simulink model "OMAP"  (R2018b)
settings: Solver=FixedStepDiscrete  StartTime=0.0  StopTime=10.0  FixedStep=0.01  RelTol=1e-3
values from neighbouring files (symbols this model uses):
  Clb_ICADirect_LaneDisp_StateFive = Simulink.Parameter    [omap_ver_442.m]
  Clb_ICADirect_LaneDisp_StateFour = Simulink.Parameter    [omap_ver_442.m]
  Clb_ICADirect_LaneDisp_StateOne = Simulink.Parameter    [omap_ver_442.m]
  Clb_ICADirect_LaneDisp_StateThree = Simulink.Parameter    [omap_ver_442.m]
  Clb_ICADirect_LaneDisp_StateTwo = Simulink.Parameter    [omap_ver_442.m]
  Clb_ICADirect_LaneDisp_StateZero = Simulink.Parameter    [omap_ver_442.m]
  Clb_ICADirect_LaneDispSW = Simulink.Parameter    [omap_ver_442.m]
  Clb_ICADirect_TrnLghtsCom_Switch = Simulink.Parameter    [omap_ver_442.m]
  Clb_ICADirect_TrnLghtsCom_Value = Simulink.Parameter    [omap_ver_442.m]
  Clb_ICADirect_TrnLghtsCrtl_Inhb = Simulink.Parameter    [omap_ver_442.m]
  OMAP_ACCAEB_EMSESC_Decel = Simulink.Parameter    [omap_ver_442.m]
  OMAP_ACCFCW_IC_Decel = Simulink.Parameter    [omap_ver_442.m]
  OMAP_clb_ACC_RVVReqType = Simulink.Parameter    [omap_ver_442.m]
  OMAP_clb_ACC_RVVReqType_Switch = Simulink.Parameter    [omap_ver_442.m]
  OMAP_clb_ACCHeadwayDisplay = Simulink.Parameter    [omap_ver_442.m]
  OMAP_clb_ACCHeadwayDisplay_Switch = Simulink.Parameter    [omap_ver_442.m]
  OMAP_clb_ACCHeadwayIcon = Simulink.Parameter    [omap_ver_442.m]
  OMAP_clb_ACCHeadwayIcon_Switch = Simulink.Parameter    [omap_ver_442.m]
  OMAP_clb_ACCMessagePrompt = Simulink.Parameter    [omap_ver_442.m]
  OMAP_clb_ACCMessagePrompt_Switch = Simulink.Parameter    [omap_ver_442.m]
  OMAP_clb_ACCRequestEPB = Simulink.Parameter    [omap_ver_442.m]
  OMAP_clb_ACCRequestEPB_Switch = Simulink.Parameter    [omap_ver_442.m]
  OMAP_clb_ACCSetSpeed = Simulink.Parameter    [omap_ver_442.m]
  OMAP_clb_ACCSetSpeed_Switch = Simulink.Parameter    [omap_ver_442.m]
  OMAP_clb_ACCSetSpeedDis = Simulink.Parameter    [omap_ver_442.m]
  OMAP_clb_ACCSetSpeedDis_Switch = Simulink.Parameter    [omap_ver_442.m]
  OMAP_clb_ACCState = Simulink.Parameter    [omap_ver_442.m]
  OMAP_clb_ACCState_Switch = Simulink.Parameter    [omap_ver_442.m]
  OMAP_clb_ACCStatusIconDis = Simulink.Parameter    [omap_ver_442.m]
  OMAP_clb_ACCStatusIconDis_Switch = Simulink.Parameter    [omap_ver_442.m]
  OMAP_clb_ACCTorqueReq = Simulink.Parameter    [omap_ver_442.m]
  OMAP_clb_ACCTorqueReq_Switch = Simulink.Parameter    [omap_ver_442.m]
  OMAP_clb_ADAS_State = Simulink.Parameter    [omap_ver_442.m]
  OMAP_clb_ADAS_State_Switch = Simulink.Parameter    [omap_ver_442.m]
  OMAP_clb_AEBAlertReq = Simulink.Parameter    [omap_ver_442.m]
  OMAP_clb_AEBAlertReq_Switch = Simulink.Parameter    [omap_ver_442.m]
  OMAP_clb_AEBBrakingProg = Simulink.Parameter    [omap_ver_442.m]
  OMAP_clb_AEBBrakingProg_Switch = Simulink.Parameter    [omap_ver_442.m]
  OMAP_clb_AEBFaultStatus = Simulink.Parameter    [omap_ver_442.m]
  OMAP_clb_AEBFaultStatus_Switch = Simulink.Parameter    [omap_ver_442.m]
  OMAP_clb_AEBMassageDisp = Simulink.Parameter    [omap_ver_442.m]
  OMAP_clb_AEBMassageDisp_Switch = Simulink.Parameter    [omap_ver_442.m]
  OMAP_clb_AEBState = Simulink.Parameter    [omap_ver_442.m]
  OMAP_clb_AEBState_Switch = Simulink.Parameter    [omap_ver_442.m]
  OMAP_clb_AEBSwitchStatus = Simulink.Parameter    [omap_ver_442.m]
  OMAP_clb_AEBSwitchStatus_Switch = Simulink.Parameter    [omap_ver_442.m]
  OMAP_clb_BrakeRequest = Simulink.Parameter    [omap_ver_442.m]
  OMAP_clb_BrakeRequest_Switch = Simulink.Parameter    [omap_ver_442.m]
  OMAP_clb_DecelerationSet = Simulink.Parameter    [omap_ver_442.m]
  OMAP_clb_DecelerationSet_Switch = Simulink.Parameter    [omap_ver_442.m]
  OMAP_clb_DecelerationType = Simulink.Parameter    [omap_ver_442.m]
  OMAP_clb_DecelerationType_Switch = Simulink.Parameter    [omap_ver_442.m]
  OMAP_clb_DeclControlReq = Simulink.Parameter    [omap_ver_442.m]
  OMAP_clb_DeclControlReq_Switch = Simulink.Parameter    [omap_ver_442.m]
  OMAP_clb_DownorUpGearMinTime = Simulink.Parameter    [omap_ver_442.m]
  OMAP_clb_DownorUpGearMinTime_Switch = Simulink.Parameter    [omap_ver_442.m]
  OMAP_clb_ELKPopupMessage = Simulink.Parameter    [omap_ver_442.m]
  OMAP_clb_ELKPopupMessage_Switch = Simulink.Parameter    [omap_ver_442.m]
  OMAP_clb_ELKSts = Simulink.Parameter    [omap_ver_442.m]
  OMAP_clb_ELKSts_Switch = Simulink.Parameter    [omap_ver_442.m]
  OMAP_clb_ESAFaultSt = Simulink.Parameter    [omap_ver_442.m]
  OMAP_clb_ESAFaultSt_Switch = Simulink.Parameter    [omap_ver_442.m]
  OMAP_clb_ESARequest = Simulink.Parameter    [omap_ver_442.m]
  OMAP_clb_ESARequest_Switch = Simulink.Parameter    [omap_ver_442.m]
  OMAP_clb_ESAState = Simulink.Parameter    [omap_ver_442.m]
  OMAP_clb_ESAState_Switch = Simulink.Parameter    [omap_ver_442.m]
  OMAP_clb_ESATorqueReq = Simulink.Parameter    [omap_ver_442.m]
  OMAP_clb_ESATorqueReq_Switch = Simulink.Parameter    [omap_ver_442.m]
  OMAP_clb_ESCDriveOff = Simulink.Parameter    [omap_ver_442.m]
  OMAP_clb_ESCDriveOff_Switch = Simulink.Parameter    [omap_ver_442.m]
  OMAP_clb_ESCHoldReq = Simulink.Parameter    [omap_ver_442.m]
  OMAP_clb_ESCHoldReq_Switch = Simulink.Parameter    [omap_ver_442.m]
  OMAP_clb_Handsoffwarning = Simulink.Parameter    [omap_ver_442.m]
  OMAP_clb_Handsoffwarning_Switch = Simulink.Parameter    [omap_ver_442.m]
  OMAP_clb_HapticAlarmReq = Simulink.Parameter    [omap_ver_442.m]
  OMAP_clb_HapticAlarmReq_Switch = Simulink.Parameter    [omap_ver_442.m]
  OMAP_clb_HMIPopupMassage = Simulink.Parameter    [omap_ver_442.m]
  OMAP_clb_HMIPopupMassage_Switch = Simulink.Parameter    [omap_ver_442.m]
  OMAP_clb_HWAActionSts = Simulink.Parameter    [omap_ver_442.m]
  OMAP_clb_HWAActionSts_Switch = Simulink.Parameter    [omap_ver_442.m]
  OMAP_clb_HWAMode = Simulink.Parameter    [omap_ver_442.m]
  OMAP_clb_HWAMode_Switch = Simulink.Parameter    [omap_ver_442.m]
  OMAP_clb_HWATurnOnIdctr = Simulink.Parameter    [omap_ver_442.m]
  OMAP_clb_HWATurnOnIdctr_Switch = Simulink.Parameter    [omap_ver_442.m]
  OMAP_clb_ICAMassageDisp = Simulink.Parameter    [omap_ver_442.m]
  OMAP_clb_ICAMassageDisp_Switch = Simulink.Parameter    [omap_ver_442.m]
  OMAP_clb_ICAStatusIcon = Simulink.Parameter    [omap_ver_442.m]
  OMAP_clb_ICAStatusIcon_Switch = Simulink.Parameter    [omap_ver_442.m]
  OMAP_clb_ISLCDriverRemind = Simulink.Parameter    [omap_ver_442.m]
  OMAP_clb_ISLCDriverRemind_Switch = Simulink.Parameter    [omap_ver_442.m]
  OMAP_clb_ISLCState = Simulink.Parameter    [omap_ver_442.m]
  OMAP_clb_ISLCState_Switch = Simulink.Parameter    [omap_ver_442.m]
  OMAP_clb_JAFaultSt = Simulink.Parameter    [omap_ver_442.m]
  OMAP_clb_JAFaultSt_Switch = Simulink.Parameter    [omap_ver_442.m]
  OMAP_clb_LCAPopupMessage = Simulink.Parameter    [omap_ver_442.m]
  OMAP_clb_LCAPopupMessage_Switch = Simulink.Parameter    [omap_ver_442.m]
  OMAP_clb_LCAStatusDisplay = Simulink.Parameter    [omap_ver_442.m]
  OMAP_clb_LCAStatusDisplay_Switch = Simulink.Parameter    [omap_ver_442.m]
  OMAP_clb_LDWStatusDisplay = Simulink.Parameter    [omap_ver_442.m]
  OMAP_clb_LDWStatusDisplay_Switch = Simulink.Parameter    [omap_ver_442.m]
  OMAP_clb_LDWWarningSt = Simulink.Parameter    [omap_ver_442.m]
  OMAP_clb_LDWWarningSt_Switch = Simulink.Parameter    [omap_ver_442.m]
  OMAP_clb_LightControlValid = Simulink.Parameter    [omap_ver_442.m]
  OMAP_clb_LightControlValid_Switch = Simulink.Parameter    [omap_ver_442.m]
  OMAP_clb_LKAActivation = Simulink.Parameter    [omap_ver_442.m]
  OMAP_clb_LKAActivation_Switch = Simulink.Parameter    [omap_ver_442.m]
  OMAP_clb_LKAAngleReq = Simulink.Parameter    [omap_ver_442.m]
  OMAP_clb_LKAAngleReq_Switch = Simulink.Parameter    [omap_ver_442.m]
  OMAP_clb_LKAMode = Simulink.Parameter    [omap_ver_442.m]
  OMAP_clb_LKAMode_Switch = Simulink.Parameter    [omap_ver_442.m]
  OMAP_clb_LKAorELK_CoolTime = Simulink.Parameter    [omap_ver_442.m]
  OMAP_clb_LKAState = Simulink.Parameter    [omap_ver_442.m]
  OMAP_clb_LKAState_Switch = Simulink.Parameter    [omap_ver_442.m]
  OMAP_clb_LKAStatusDisplay = Simulink.Parameter    [omap_ver_442.m]
  OMAP_clb_LKAStatusDisplay_Switch = Simulink.Parameter    [omap_ver_442.m]
  OMAP_clb_LKASwitchState = Simulink.Parameter    [omap_ver_442.m]
  OMAP_clb_LKASwitchState_Switch = Simulink.Parameter    [omap_ver_442.m]
  OMAP_clb_LKATorqFactReq = Simulink.Parameter    [omap_ver_442.m]
  OMAP_clb_LKATorqFactReq_Switch = Simulink.Parameter    [omap_ver_442.m]
  OMAP_clb_PrefillRequest = Simulink.Parameter    [omap_ver_442.m]
  ... (+36 more)
libraries: simulink x184, canmsglib x2
(part 2 of 14)

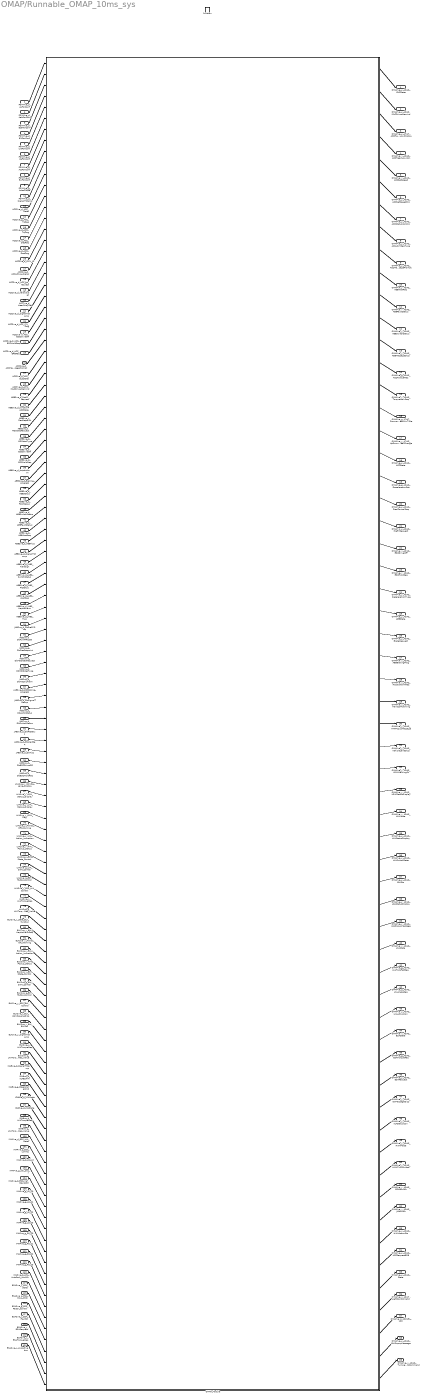
== system OMAP/Runnable_OMAP_10ms_sys ==
  FDMMve_d_JaFcnConf : Inport  OutDataTypeStr=uint16  PortDimensions=1
  FDMMve_d_AebFcnConf : Inport  Port=2  OutDataTypeStr=uint16  PortDimensions=1
  FDMMve_d_EsaFcnConf : Inport  Port=3  OutDataTypeStr=uint16  PortDimensions=1
  FDMMve_d_ElkFcnConf : Inport  Port=4  OutDataTypeStr=uint16  PortDimensions=1
  FDMMve_d_LkaFcnConf : Inport  Port=5  OutDataTypeStr=uint16  PortDimensions=1
  FDMMve_d_IcaFcnConf : Inport  Port=6  OutDataTypeStr=uint16  PortDimensions=1
  FDMMve_d_AccFcnConf : Inport  Port=7  OutDataTypeStr=uint16  PortDimensions=1
  FDMMve_d_EwFcnConf : Inport  Port=8  OutDataTypeStr=uint16  PortDimensions=1
  FDMMve_g_Adas2Fapa : Inport  Port=9  OutDataTypeStr=uint32  PortDimensions=1
  FDMMve_d_SignalTStamp : Inport  Port=10  OutDataTypeStr=uint16  PortDimensions=1
  ACCSve_d_ACC_State : Inport  Port=11  OutDataTypeStr=uint16  PortDimensions=1
  ACCSve_g_ACC_TqReq : Inport  Port=12  OutDataTypeStr=single  PortDimensions=1
  ACCSve_d_ACC_TqFlag : Inport  Port=13  OutDataTypeStr=uint16  PortDimensions=1
  ACCSve_g_ACC_DecReq : Inport  Port=14  OutDataTypeStr=single  PortDimensions=1
  ACCSve_d_ACC_DecFlag : Inport  Port=15  OutDataTypeStr=uint16  PortDimensions=1
  ACCSve_d_CIPV_ID : Inport  Port=16  OutDataTypeStr=uint16  PortDimensions=1
  ACCSve_d_ACCActive_Signal : Inport  Port=17  OutDataTypeStr=uint16  PortDimensions=1
  ACCSve_d_ACC_go_request : Inport  Port=18  OutDataTypeStr=uint16  PortDimensions=1
  ACCSve_d_VelocitySet : Inport  Port=19  OutDataTypeStr=uint16  PortDimensions=1
  ACCSve_d_HeadWaySet : Inport  Port=20  OutDataTypeStr=uint16  PortDimensions=1
  ACCSve_d_SignalTStamp : Inport  Port=21  OutDataTypeStr=uint16  PortDimensions=1
  ACCSve_d_ACC_ICA_Flag : Inport  Port=22  OutDataTypeStr=uint16  PortDimensions=1
  ACCSve_d_ACC_ESCDriveOff : Inport  Port=23  OutDataTypeStr=uint16  PortDimensions=1
  ACCSve_d_ACC_ESCHoldReq : Inport  Port=24  OutDataTypeStr=uint16  PortDimensions=1
  ACCSve_d_ACC_EPBReq : Inport  Port=25  OutDataTypeStr=uint16  PortDimensions=1
  ACCSve_d_ACCMessagePrompt : Inport  Port=26  OutDataTypeStr=uint16
  ACCSve_d_ACC_ISLCState : Inport  Port=27  OutDataTypeStr=uint16  PortDimensions=1
  ACCSve_d_ACC_ISLCDriverRemind : Inport  Port=28  OutDataTypeStr=uint16  PortDimensions=1
  AEBSve_d_Prefill_request : Inport  Port=29  OutDataTypeStr=uint16  PortDimensions=1
  AEBSve_d_functionFARCState : Inport  Port=30  OutDataTypeStr=uint16  PortDimensions=1
  AEBSve_g_DecSetpoint : Inport  Port=31  OutDataTypeStr=single  PortDimensions=1
  AEBSve_d_MDDdecRequest : Inport  Port=32  OutDataTypeStr=uint16  PortDimensions=1
  AEBSve_d_MDDdecType : Inport  Port=33  OutDataTypeStr=uint16  PortDimensions=1
  AEBSve_d_ESCDriveOff : Inport  Port=34  OutDataTypeStr=uint16  PortDimensions=1
  AEBSve_d_ESCHoldReq : Inport  Port=35  OutDataTypeStr=uint16  PortDimensions=1
  AEBSve_d_HapticAlarm : Inport  Port=36  OutDataTypeStr=uint16  PortDimensions=1
  AEBSve_d_Braking_progress : Inport  Port=37  OutDataTypeStr=uint16  PortDimensions=1
  AEBSve_d_AEBStatus : Inport  Port=38  OutDataTypeStr=uint16  PortDimensions=1
  AEBSve_d_FCWStatus : Inport  Port=39  OutDataTypeStr=uint16  PortDimensions=1
  AEBSve_d_AEBSwitchStatus : Inport  Port=40  OutDataTypeStr=uint16  PortDimensions=1
  AEBSve_d_AEBFaultStatus : Inport  Port=41  OutDataTypeStr=uint16  PortDimensions=1
  AEBSve_d_AEBAlertReq : Inport  Port=42  OutDataTypeStr=uint16  PortDimensions=1
  AEBSve_d_AEBTips : Inport  Port=43  OutDataTypeStr=uint16  PortDimensions=1
  AEBSve_d_SignalTStamp : Inport  Port=44  OutDataTypeStr=uint16  PortDimensions=1
  AEBSve_d_JABS_AlertSign : Inport  Port=45  OutDataTypeStr=uint16  PortDimensions=1
  AEBSve_d_JABS_SwitchStatus : Inport  Port=46  OutDataTypeStr=uint16  PortDimensions=1
  AEBSve_d_JABS_FltStatus : Inport  Port=47  OutDataTypeStr=uint16  PortDimensions=1
  AEBSve_d_JABS_AlertReq : Inport  Port=48  OutDataTypeStr=uint16  PortDimensions=1
  AEBSve_d_JABS_HapticAlarm : Inport  Port=49  OutDataTypeStr=uint16  PortDimensions=1
  AEBSve_d_JABS_Tips : Inport  Port=50  OutDataTypeStr=uint16  PortDimensions=1
  JABSve_d_DbPrefillReq : Inport  Port=51  OutDataTypeStr=uint16  PortDimensions=1
  JABSve_d_DbFunFARCSta : Inport  Port=52  OutDataTypeStr=uint16  PortDimensions=1
  JABSve_g_DbDecSetpoint : Inport  Port=53  OutDataTypeStr=single  PortDimensions=1
  JABSve_d_DbMDDdecRequest : Inport  Port=54  OutDataTypeStr=uint16  PortDimensions=1
  JABSve_d_DbMDDdecType : Inport  Port=55  OutDataTypeStr=uint16  PortDimensions=1
  JABSve_d_DbHapticAlarm : Inport  Port=56  OutDataTypeStr=uint16  PortDimensions=1
  JABSve_d_DbBraking_progress : Inport  Port=57  OutDataTypeStr=uint16  PortDimensions=1
  JABSve_d_DbSignalTStamp : Inport  Port=58  OutDataTypeStr=uint16  PortDimensions=1
  JABSve_d_DbJACWStatus : Inport  Port=59  OutDataTypeStr=uint16  PortDimensions=1
  JABSve_d_DbSwitchStatus : Inport  Port=60  OutDataTypeStr=uint16  PortDimensions=1
  JABSve_d_DbFltStatus : Inport  Port=61  OutDataTypeStr=uint16  PortDimensions=1
  JABSve_d_DbAlertReq : Inport  Port=62  OutDataTypeStr=uint16  PortDimensions=1
  JABSve_d_DbTips : Inport  Port=63  OutDataTypeStr=uint16  PortDimensions=1
  JABSve_d_DbESCDriveOff : Inport  Port=64  OutDataTypeStr=uint16  PortDimensions=1
  JABSve_d_DbESCHoldReq : Inport  Port=65  OutDataTypeStr=uint16  PortDimensions=1
  LKASve_y_Vehicle_Lane_Display : Inport  Port=66  OutDataTypeStr=uint8  PortDimensions=1
  LKASve_y_LDW_Status_Display : Inport  Port=67  OutDataTypeStr=uint8  PortDimensions=1
  LKASve_y_LKA_Status_Display : Inport  Port=68  OutDataTypeStr=uint8  PortDimensions=1
  LKASve_y_LDW_Flag : Inport  Port=69  OutDataTypeStr=uint8  PortDimensions=1
  LKASve_y_Hands_Off_Warning : Inport  Port=70  OutDataTypeStr=uint8  PortDimensions=1
  LKASve_y_LKA_Action_Indication : Inport  Port=71  OutDataTypeStr=uint8  PortDimensions=1
  LKASve_y_HMI_Popup_Status : Inport  Port=72  OutDataTypeStr=uint8  PortDimensions=1
  LKASve_y_EPS_State_Control : Inport  Port=73  OutDataTypeStr=uint8  PortDimensions=1
  LKASve_g_LKA_SWA_Control : Inport  Port=74  OutDataTypeStr=single  PortDimensions=1
  LKASve_g_EPS_Factor_Control : Inport  Port=75  OutDataTypeStr=single  PortDimensions=1
  LKASve_y_EPS_LKA_Control : Inport  Port=76  OutDataTypeStr=uint8  PortDimensions=1
  LKASve_y_LKATorqueReq : Inport  Port=77  OutDataTypeStr=uint8  PortDimensions=1
  LKASve_g_LKATorqueReq_Value : Inport  Port=78  OutDataTypeStr=single  PortDimensions=1
  ELKSve_y_state_ELK_function : Inport  Port=79  OutDataTypeStr=uint8  PortDimensions=1
  ELKSve_y_ELK_HapticAlarmReq : Inport  Port=80  OutDataTypeStr=uint8  PortDimensions=1
  ELKSve_y_Hands_Off_Warning : Inport  Port=81  OutDataTypeStr=uint8  PortDimensions=1
  ELKSve_y_ELK_Action_Indication : Inport  Port=82  OutDataTypeStr=uint8  PortDimensions=1
  ELKSve_y_HMI_Popup_Status : Inport  Port=83  OutDataTypeStr=uint8  PortDimensions=1
  ELKSve_y_EPS_State_Control : Inport  Port=84  OutDataTypeStr=uint8  PortDimensions=1
  ELKSve_g_ELK_SWA_Control : Inport  Port=85  OutDataTypeStr=single  PortDimensions=1
  ELKSve_g_EPS_Factor_Control : Inport  Port=86  OutDataTypeStr=single  PortDimensions=1
  ELKSve_y_EPS_ELK_Control : Inport  Port=87  OutDataTypeStr=uint8  PortDimensions=1
  ELKSve_y_ELK_VehicleLaneDisp : Inport  Port=88  OutDataTypeStr=uint8  PortDimensions=1
  ELKSve_y_ELK_ELKSts : Inport  Port=89  OutDataTypeStr=uint8  PortDimensions=1
  ELKSve_y_SignalTStamp : Inport  Port=90  OutDataTypeStr=uint8  PortDimensions=1
  ELKSve_y_LKATorqueReq : Inport  Port=91  OutDataTypeStr=uint8  PortDimensions=1
  ELKSve_g_LKATorqueReq_Value : Inport  Port=92  OutDataTypeStr=single  PortDimensions=1
  ICABve_d_SignalTStamp : Inport  Port=93  OutDataTypeStr=uint16  PortDimensions=1
  ICABva_d_ICAB2HMI : Inport  Port=94  OutDataTypeStr=uint16  PortDimensions=20
  ICABve_g_SteerAngleCmd : Inport  Port=95  OutDataTypeStr=single  PortDimensions=1
  ICABve_d_ICAMode : Inport  Port=96  OutDataTypeStr=uint16  PortDimensions=1
  ICABve_d_ICAState : Inport  Port=97  OutDataTypeStr=uint16  PortDimensions=1
  ICABve_d_LKATorqueReq : Inport  Port=98  OutDataTypeStr=uint16  PortDimensions=1
  ICABve_g_LKATorqueReq_Value : Inport  Port=99  OutDataTypeStr=single  PortDimensions=1
  IMAPve_d_EPS_LKA_State : Inport  Port=100  OutDataTypeStr=uint16  PortDimensions=1
  IMAPve_g_ESC_LonAcc : Inport  Port=101  OutDataTypeStr=single  PortDimensions=1
  IMAPva_d_obj_id : Inport  Port=102  OutDataTypeStr=uint16  PortDimensions=40
  IMAPva_g_obj_pos_x : Inport  Port=103  OutDataTypeStr=single  PortDimensions=40
  IMAPve_d_ESC_Veh_Standstill : Inport  Port=104  OutDataTypeStr=uint16  PortDimensions=1
  IMAPve_g_L0_C0 : Inport  Port=105  OutDataTypeStr=single  PortDimensions=1
  IMAPve_g_L0_C1 : Inport  Port=106  OutDataTypeStr=single  PortDimensions=1
  IMAPve_g_L0_C2 : Inport  Port=107  OutDataTypeStr=single  PortDimensions=1
  IMAPve_g_L0_C3 : Inport  Port=108  OutDataTypeStr=single  PortDimensions=1
  IMAPve_g_R0_C0 : Inport  Port=109  OutDataTypeStr=single  PortDimensions=1
  IMAPve_g_R0_C1 : Inport  Port=110  OutDataTypeStr=single  PortDimensions=1
  IMAPve_g_R0_C2 : Inport  Port=111  OutDataTypeStr=single  PortDimensions=1
  IMAPve_g_R0_C3 : Inport  Port=112  OutDataTypeStr=single  PortDimensions=1
  IMAPve_d_APA_AutoPark_WorkSt : Inport  Port=113  OutDataTypeStr=uint16  PortDimensions=1
  ESASve_y_ESA_State : Inport  Port=114  OutDataTypeStr=uint8
  ESASve_g_ESA_SWA_CMD : Inport  Port=115  OutDataTypeStr=single
  ESASve_g_EPS_Factor_Control : Inport  Port=116  OutDataTypeStr=single
  ESASve_y_ESA_FaultSt : Inport  Port=117  OutDataTypeStr=uint8
  ESASve_y_ESARequest : Inport  Port=118  OutDataTypeStr=uint8
  ESASve_y_ESATorqueReq : Inport  Port=119  OutDataTypeStr=single
  ESASve_y_LKAActivation : Inport  Port=120  OutDataTypeStr=uint8
  function : TriggerPort  TriggerType=function-call  VariantControl=Variant  SampleTimeType=periodic  SampleTime=-1
  OMAP_Module : Subsystem  TreatAsAtomicUnit=on
  OMAPve_y_ADAS_ISLCState : Outport  OutDataTypeStr=uint8  PortDimensions=1
  OMAPve_y_ADAS_ISLCDriverRemind : Outport  Port=2  OutDataTypeStr=uint8  PortDimensions=1
  OMAPve_y_ADAS_ACCHeadwayDisplay : Outport  Port=3  OutDataTypeStr=uint8  PortDimensions=1
  OMAPve_y_ADAS_ACCHeadwayIcon : Outport  Port=4  OutDataTypeStr=uint8  PortDimensions=1
  OMAPve_y_ADAS_ACCSetSpeed : Outport  Port=5  OutDataTypeStr=uint8  PortDimensions=1
  OMAPve_y_ADAS_ACCSetSpeedDis : Outport  Port=6  OutDataTypeStr=uint8  PortDimensions=1
  OMAPve_y_ADAS_ACCStatusIconDis : Outport  Port=7  OutDataTypeStr=uint8  PortDimensions=1
  OMAPve_y_ADAS_ACC_RVVReqType : Outport  Port=8  OutDataTypeStr=uint8  PortDimensions=1
  OMAPve_y_ADAS_ACCMessagePrompt : Outport  Port=9  OutDataTypeStr=uint8  PortDimensions=1
  OMAPve_y_ADAS_AEBAlertReq : Outport  Port=10  OutDataTypeStr=uint8  PortDimensions=1
  OMAPve_y_ADAS_AEBFaultStatus : Outport  Port=11  OutDataTypeStr=uint8  PortDimensions=1
  OMAPve_y_ADAS_AEBSwitchStatus : Outport  Port=12  OutDataTypeStr=uint8  PortDimensions=1
  OMAPve_y_ADAS_AEBMassageDisp : Outport  Port=13  OutDataTypeStr=uint8  PortDimensions=1
  OMAPve_g_ADAS_ACCTorqueReq : Outport  Port=14  OutDataTypeStr=single  PortDimensions=1
  OMAPve_y_ADAS_TorqueActivReq : Outport  Port=15  OutDataTypeStr=uint8  PortDimensions=1
  OMAPve_g_ADAS_DownorUpGearMinTime : Outport  Port=16  OutDataTypeStr=single  PortDimensions=1
  OMAPve_y_ADAS_UpDownGearChange : Outport  Port=17  OutDataTypeStr=uint8  PortDimensions=1
  OMAPve_y_ADAS_ACCState : Outport  Port=18  OutDataTypeStr=uint8  PortDimensions=1
  OMAPve_g_ADAS_DecelerationSet : Outport  Port=19  OutDataTypeStr=single  PortDimensions=1
  OMAPve_y_ADAS_DeclControlReq : Outport  Port=20  OutDataTypeStr=uint8  PortDimensions=1
  OMAPve_y_ADAS_PrefillRequest : Outport  Port=21  OutDataTypeStr=uint8  PortDimensions=1
  OMAPve_y_ADAS_ESCDriveOff : Outport  Port=22  OutDataTypeStr=uint8  PortDimensions=1
  OMAPve_y_ADAS_ESCHoldReq : Outport  Port=23  OutDataTypeStr=uint8  PortDimensions=1
  OMAPve_y_ADAS_DecelerationType : Outport  Port=24  OutDataTypeStr=uint8  PortDimensions=1
  OMAPve_y_ADAS_AEBState : Outport  Port=25  OutDataTypeStr=uint8  PortDimensions=1
  OMAPve_y_ADAS_BrakeRequest : Outport  Port=26  OutDataTypeStr=uint8  PortDimensions=1
  OMAPve_y_ADAS_AEBBrakingProg : Outport  Port=27  OutDataTypeStr=uint8  PortDimensions=1
  OMAPve_y_ADAS_HapticAlarmReq : Outport  Port=28  OutDataTypeStr=uint8  PortDimensions=1
  OMAPve_y_ADAS_Handsoffwarning : Outport  Port=29  OutDataTypeStr=uint8  PortDimensions=1
  OMAPve_y_ADAS_HMIPopupMassage : Outport  Port=30  OutDataTypeStr=uint8  PortDimensions=1
  OMAPve_y_ADAS_VehicleLaneDisp : Outport  Port=31  OutDataTypeStr=uint8  PortDimensions=1
  OMAPve_y_ADAS_LDWWarningSt : Outport  Port=32  OutDataTypeStr=uint8  PortDimensions=1
  OMAPve_y_ADAS_LDWStatusDisplay : Outport  Port=33  OutDataTypeStr=uint8  PortDimensions=1
  OMAPve_y_ADAS_LKAMode : Outport  Port=34  OutDataTypeStr=uint8  PortDimensions=1
  OMAPve_y_ADAS_LKAStatusDisplay : Outport  Port=35  OutDataTypeStr=uint8  PortDimensions=1
  OMAPve_y_ADAS_LKASwitchState : Outport  Port=36  OutDataTypeStr=uint8  PortDimensions=1
  OMAPve_y_ADAS_ELKSts : Outport  Port=37  OutDataTypeStr=uint8  PortDimensions=1
  OMAPve_y_ADAS_LCAStatusDisplay : Outport  Port=38  OutDataTypeStr=uint8  PortDimensions=1
  OMAPve_y_ADAS_LCAPopupMessage : Outport  Port=39  OutDataTypeStr=uint8  PortDimensions=1
  OMAPve_y_ADAS_LKAState : Outport  Port=40  OutDataTypeStr=uint8  PortDimensions=1
  OMAPve_g_ADAS_LKATorqFactReq : Outport  Port=41  OutDataTypeStr=single  PortDimensions=1
  OMAPve_g_ADAS_LKAAngleReq : Outport  Port=42  OutDataTypeStr=single  PortDimensions=1
  OMAPve_y_ADAS_LKAActivation : Outport  Port=43  OutDataTypeStr=uint8  PortDimensions=1
  OMAPve_y_ADAS_ESAState : Outport  Port=44  OutDataTypeStr=uint8  PortDimensions=1
  OMAPve_g_ADAS_ESATorqueReq : Outport  Port=45  OutDataTypeStr=single  PortDimensions=1
  OMAPve_y_ADAS_ESARequest : Outport  Port=46  OutDataTypeStr=uint8  PortDimensions=1
  OMAPve_y_ADAS_ICAMassageDisp : Outport  Port=47  OutDataTypeStr=uint8  PortDimensions=1
  OMAPve_y_ADAS_ICAStatusIcon : Outport  Port=48  OutDataTypeStr=uint8  PortDimensions=1
  OMAPve_y_ADAS_HWAMode : Outport  Port=49  OutDataTypeStr=uint8  PortDimensions=1
  OMAPve_y_ADAS_HWATurnOnIdctr : Outport  Port=50  OutDataTypeStr=uint8  PortDimensions=1
  OMAPve_y_ADAS_ESAFaultSt : Outport  Port=51  OutDataTypeStr=uint8  PortDimensions=1
  OMAPve_y_ADAS_JAFaultSt : Outport  Port=52  OutDataTypeStr=uint8  PortDimensions=1
  OMAPve_y_ADAS_HWAActionSts : Outport  Port=53  OutDataTypeStr=uint8  PortDimensions=1
  OMAPve_y_ADAS_ACCRequestEPB : Outport  Port=54  OutDataTypeStr=uint8  PortDimensions=1
  OMAPve_y_ADAS_State : Outport  Port=55  OutDataTypeStr=uint8  PortDimensions=1
  OMAPve_y_ADAS_LightControlValid : Outport  Port=56  OutDataTypeStr=uint8  PortDimensions=1
  OMAPve_g_ob019L_100 : Outport  Port=57  OutDataTypeStr=uint32  PortDimensions=1
  OMAPve_y_ADAS_ELKPopupMessage : Outport  Port=58  OutDataTypeStr=uint8
  OMAPve_y_ADAS_TurnLightsCommand : Outport  Port=59  OutDataTypeStr=uint8
  wires:
  ELKSve_y_HMI_Popup_Status/1 -> OMAP_Module/83(ELKSve_y_HMI_Popup_Status)
  FDMMve_d_ElkFcnConf/1 -> OMAP_Module/4(FDMMve_d_ElkFcnConf)
  AEBSve_d_AEBFaultStatus/1 -> OMAP_Module/41(AEBSve_d_AEBFaultStatus)
  OMAP_Module/36(OMAPve_y_ADAS_LKASwitchState) -> OMAPve_y_ADAS_LKASwitchState/1
  AEBSve_d_Braking_progress/1 -> OMAP_Module/37(AEBSve_d_Braking_progress)
  OMAP_Module/9(OMAPve_y_ADAS_ACCMessagePrompt) -> OMAPve_y_ADAS_ACCMessagePrompt/1
  OMAP_Module/31(OMAPve_y_ADAS_VehicleLaneDisp) -> OMAPve_y_ADAS_VehicleLaneDisp/1
  FDMMve_d_AebFcnConf/1 -> OMAP_Module/2(FDMMve_d_AebFcnConf)
  ACCSve_d_ACC_DecFlag/1 -> OMAP_Module/15(ACCSve_d_ACC_DecFlag)
  ICABva_d_ICAB2HMI/1 -> OMAP_Module/94(ICABva_d_ICAB2HMI)
  OMAP_Module/32(OMAPve_y_ADAS_LDWWarningSt) -> OMAPve_y_ADAS_LDWWarningSt/1
  AEBSve_d_AEBStatus/1 -> OMAP_Module/38(AEBSve_d_AEBStatus)
  IMAPve_d_ESC_Veh_Standstill/1 -> OMAP_Module/104(IMAPve_d_ESC_Veh_Standstill)
  FDMMve_g_Adas2Fapa/1 -> OMAP_Module/9(FDMMve_g_Adas2Fapa)
  OMAP_Module/41(OMAPve_g_ADAS_LKATorqFactReq) -> OMAPve_g_ADAS_LKATorqFactReq/1
  ELKSve_g_ELK_SWA_Control/1 -> OMAP_Module/85(ELKSve_g_ELK_SWA_Control)
  FDMMve_d_IcaFcnConf/1 -> OMAP_Module/6(FDMMve_d_IcaFcnConf)
  LKASve_y_EPS_State_Control/1 -> OMAP_Module/73(LKASve_y_EPS_State_Control)
  OMAP_Module/14(OMAPve_g_ADAS_ACCTorqueReq) -> OMAPve_g_ADAS_ACCTorqueReq/1
  ELKSve_y_ELK_ELKSts/1 -> OMAP_Module/89(ELKSve_y_ELK_ELKSts)
  ICABve_d_SignalTStamp/1 -> OMAP_Module/93(ICABve_d_SignalTStamp)
  AEBSve_d_MDDdecRequest/1 -> OMAP_Module/32(AEBSve_d_MDDdecRequest)
  ELKSve_y_state_ELK_function/1 -> OMAP_Module/79(ELKSve_y_state_ELK_function)
  OMAP_Module/6(OMAPve_y_ADAS_ACCSetSpeedDis) -> OMAPve_y_ADAS_ACCSetSpeedDis/1
  ACCSve_d_ACCActive_Signal/1 -> OMAP_Module/17(ACCSve_d_ACCActive_Signal)
  AEBSve_g_DecSetpoint/1 -> OMAP_Module/31(AEBSve_g_DecSetpoint)
  IMAPve_g_L0_C2/1 -> OMAP_Module/107(IMAPve_g_L0_C2)
  JABSve_d_DbSwitchStatus/1 -> OMAP_Module/60(JABSve_d_DbSwitchStatus)
  ACCSve_d_VelocitySet/1 -> OMAP_Module/19(ACCSve_d_VelocitySet)
  ELKSve_y_SignalTStamp/1 -> OMAP_Module/90(ELKSve_y_SignalTStamp)
  ACCSve_d_ACC_ICA_Flag/1 -> OMAP_Module/22(ACCSve_d_ACC_ICA_Flag)
  AEBSve_d_AEBAlertReq/1 -> OMAP_Module/42(AEBSve_d_AEBAlertReq)
  JABSve_d_DbMDDdecType/1 -> OMAP_Module/55(JABSve_d_DbMDDdecType)
  OMAP_Module/13(OMAPve_y_ADAS_AEBMassageDisp) -> OMAPve_y_ADAS_AEBMassageDisp/1
  LKASve_y_EPS_LKA_Control/1 -> OMAP_Module/76(LKASve_y_EPS_LKA_Control)
  ELKSve_y_ELK_Action_Indication/1 -> OMAP_Module/82(ELKSve_y_ELK_Action_Indication)
  AEBSve_d_JABS_FltStatus/1 -> OMAP_Module/47(AEBSve_d_JABS_FltStatus)
  OMAP_Module/47(OMAPve_y_ADAS_ICAMassageDisp) -> OMAPve_y_ADAS_ICAMassageDisp/1
  OMAP_Module/4(OMAPve_y_ADAS_ACCHeadwayIcon) -> OMAPve_y_ADAS_ACCHeadwayIcon/1
  OMAP_Module/8(OMAPve_y_ADAS_ACC_RVVReqType) -> OMAPve_y_ADAS_ACC_RVVReqType/1
  JABSve_d_DbPrefillReq/1 -> OMAP_Module/51(JABSve_d_DbPrefillReq)
  LKASve_y_LDW_Status_Display/1 -> OMAP_Module/67(LKASve_y_LDW_Status_Display)
  AEBSve_d_JABS_Tips/1 -> OMAP_Module/50(AEBSve_d_JABS_Tips)
  AEBSve_d_JABS_AlertReq/1 -> OMAP_Module/48(AEBSve_d_JABS_AlertReq)
  AEBSve_d_JABS_AlertSign/1 -> OMAP_Module/45(AEBSve_d_JABS_AlertSign)
  OMAP_Module/11(OMAPve_y_ADAS_AEBFaultStatus) -> OMAPve_y_ADAS_AEBFaultStatus/1
  AEBSve_d_FCWStatus/1 -> OMAP_Module/39(AEBSve_d_FCWStatus)
  JABSve_d_DbFunFARCSta/1 -> OMAP_Module/52(JABSve_d_DbFunFARCSta)
  AEBSve_d_SignalTStamp/1 -> OMAP_Module/44(AEBSve_d_SignalTStamp)
  ELKSve_g_EPS_Factor_Control/1 -> OMAP_Module/86(ELKSve_g_EPS_Factor_Control)
  IMAPve_g_R0_C1/1 -> OMAP_Module/110(IMAPve_g_R0_C1)
  JABSve_d_DbTips/1 -> OMAP_Module/63(JABSve_d_DbTips)
  AEBSve_d_functionFARCState/1 -> OMAP_Module/30(AEBSve_d_functionFARCState)
  JABSve_d_DbBraking_progress/1 -> OMAP_Module/57(JABSve_d_DbBraking_progress)
  AEBSve_d_MDDdecType/1 -> OMAP_Module/33(AEBSve_d_MDDdecType)
  LKASve_y_Vehicle_Lane_Display/1 -> OMAP_Module/66(LKASve_y_Vehicle_Lane_Display)
  AEBSve_d_HapticAlarm/1 -> OMAP_Module/36(AEBSve_d_HapticAlarm)
  OMAP_Module/12(OMAPve_y_ADAS_AEBSwitchStatus) -> OMAPve_y_ADAS_AEBSwitchStatus/1
  OMAP_Module/5(OMAPve_y_ADAS_ACCSetSpeed) -> OMAPve_y_ADAS_ACCSetSpeed/1
  ELKSve_y_EPS_State_Control/1 -> OMAP_Module/84(ELKSve_y_EPS_State_Control)
  OMAP_Module/26(OMAPve_y_ADAS_BrakeRequest) -> OMAPve_y_ADAS_BrakeRequest/1
  AEBSve_d_ESCHoldReq/1 -> OMAP_Module/35(AEBSve_d_ESCHoldReq)
  OMAP_Module/21(OMAPve_y_ADAS_PrefillRequest) -> OMAPve_y_ADAS_PrefillRequest/1
  OMAP_Module/43(OMAPve_y_ADAS_LKAActivation) -> OMAPve_y_ADAS_LKAActivation/1
  ACCSve_g_ACC_DecReq/1 -> OMAP_Module/14(ACCSve_g_ACC_DecReq)
  ACCSve_g_ACC_TqReq/1 -> OMAP_Module/12(ACCSve_g_ACC_TqReq)
  OMAP_Module/10(OMAPve_y_ADAS_AEBAlertReq) -> OMAPve_y_ADAS_AEBAlertReq/1
  OMAP_Module/50(OMAPve_y_ADAS_HWATurnOnIdctr) -> OMAPve_y_ADAS_HWATurnOnIdctr/1
  JABSve_d_DbSignalTStamp/1 -> OMAP_Module/58(JABSve_d_DbSignalTStamp)
  ELKSve_y_EPS_ELK_Control/1 -> OMAP_Module/87(ELKSve_y_EPS_ELK_Control)
  IMAPve_g_L0_C0/1 -> OMAP_Module/105(IMAPve_g_L0_C0)
  IMAPva_d_obj_id/1 -> OMAP_Module/102(IMAPva_d_obj_id)
  OMAP_Module/2(OMAPve_y_ADAS_ISLCDriverRemind) -> OMAPve_y_ADAS_ISLCDriverRemind/1
  JABSve_d_DbHapticAlarm/1 -> OMAP_Module/56(JABSve_d_DbHapticAlarm)
  AEBSve_d_AEBTips/1 -> OMAP_Module/43(AEBSve_d_AEBTips)
  IMAPve_g_R0_C3/1 -> OMAP_Module/112(IMAPve_g_R0_C3)
  ACCSve_d_CIPV_ID/1 -> OMAP_Module/16(ACCSve_d_CIPV_ID)
  OMAP_Module/27(OMAPve_y_ADAS_AEBBrakingProg) -> OMAPve_y_ADAS_AEBBrakingProg/1
  LKASve_y_LKA_Action_Indication/1 -> OMAP_Module/71(LKASve_y_LKA_Action_Indication)
  OMAP_Module/3(OMAPve_y_ADAS_ACCHeadwayDisplay) -> OMAPve_y_ADAS_ACCHeadwayDisplay/1
  ACCSve_d_ACC_go_request/1 -> OMAP_Module/18(ACCSve_d_ACC_go_request)
  IMAPve_g_L0_C1/1 -> OMAP_Module/106(IMAPve_g_L0_C1)
  LKASve_g_EPS_Factor_Control/1 -> OMAP_Module/75(LKASve_g_EPS_Factor_Control)
  OMAP_Module/22(OMAPve_y_ADAS_ESCDriveOff) -> OMAPve_y_ADAS_ESCDriveOff/1
  JABSve_d_DbMDDdecRequest/1 -> OMAP_Module/54(JABSve_d_DbMDDdecRequest)
  OMAP_Module/38(OMAPve_y_ADAS_LCAStatusDisplay) -> OMAPve_y_ADAS_LCAStatusDisplay/1
  OMAP_Module/28(OMAPve_y_ADAS_HapticAlarmReq) -> OMAPve_y_ADAS_HapticAlarmReq/1
  FDMMve_d_AccFcnConf/1 -> OMAP_Module/7(FDMMve_d_AccFcnConf)
  JABSve_d_DbESCHoldReq/1 -> OMAP_Module/65(JABSve_d_DbESCHoldReq)
  OMAP_Module/25(OMAPve_y_ADAS_AEBState) -> OMAPve_y_ADAS_AEBState/1
  OMAP_Module/16(OMAPve_g_ADAS_DownorUpGearMinTime) -> OMAPve_g_ADAS_DownorUpGearMinTime/1
  OMAP_Module/20(OMAPve_y_ADAS_DeclControlReq) -> OMAPve_y_ADAS_DeclControlReq/1
  OMAP_Module/29(OMAPve_y_ADAS_Handsoffwarning) -> OMAPve_y_ADAS_Handsoffwarning/1
  OMAP_Module/53(OMAPve_y_ADAS_HWAActionSts) -> OMAPve_y_ADAS_HWAActionSts/1
  OMAP_Module/15(OMAPve_y_ADAS_TorqueActivReq) -> OMAPve_y_ADAS_TorqueActivReq/1
  OMAP_Module/30(OMAPve_y_ADAS_HMIPopupMassage) -> OMAPve_y_ADAS_HMIPopupMassage/1
  IMAPve_g_ESC_LonAcc/1 -> OMAP_Module/101(IMAPve_g_ESC_LonAcc)
  AEBSve_d_Prefill_request/1 -> OMAP_Module/29(AEBSve_d_Prefill_request)
  ACCSve_d_ACC_ESCDriveOff/1 -> OMAP_Module/23(ACCSve_d_ACC_ESCDriveOff)
  IMAPve_g_R0_C0/1 -> OMAP_Module/109(IMAPve_g_R0_C0)
  OMAP_Module/34(OMAPve_y_ADAS_LKAMode) -> OMAPve_y_ADAS_LKAMode/1
  OMAP_Module/44(OMAPve_y_ADAS_ESAState) -> OMAPve_y_ADAS_ESAState/1
  OMAP_Module/33(OMAPve_y_ADAS_LDWStatusDisplay) -> OMAPve_y_ADAS_LDWStatusDisplay/1
  LKASve_y_LDW_Flag/1 -> OMAP_Module/69(LKASve_y_LDW_Flag)
  ELKSve_y_ELK_VehicleLaneDisp/1 -> OMAP_Module/88(ELKSve_y_ELK_VehicleLaneDisp)
  OMAP_Module/18(OMAPve_y_ADAS_ACCState) -> OMAPve_y_ADAS_ACCState/1
  OMAP_Module/52(OMAPve_y_ADAS_JAFaultSt) -> OMAPve_y_ADAS_JAFaultSt/1
  JABSve_d_DbFltStatus/1 -> OMAP_Module/61(JABSve_d_DbFltStatus)
  OMAP_Module/56(OMAPve_y_ADAS_LightControlValid) -> OMAPve_y_ADAS_LightControlValid/1
  ACCSve_d_ACC_ESCHoldReq/1 -> OMAP_Module/24(ACCSve_d_ACC_ESCHoldReq)
  OMAP_Module/54(OMAPve_y_ADAS_ACCRequestEPB) -> OMAPve_y_ADAS_ACCRequestEPB/1
  OMAP_Module/37(OMAPve_y_ADAS_ELKSts) -> OMAPve_y_ADAS_ELKSts/1
  LKASve_y_HMI_Popup_Status/1 -> OMAP_Module/72(LKASve_y_HMI_Popup_Status)
  OMAP_Module/7(OMAPve_y_ADAS_ACCStatusIconDis) -> OMAPve_y_ADAS_ACCStatusIconDis/1
  FDMMve_d_EwFcnConf/1 -> OMAP_Module/8(FDMMve_d_EwFcnConf)
  JABSve_d_DbJACWStatus/1 -> OMAP_Module/59(JABSve_d_DbJACWStatus)
  JABSve_g_DbDecSetpoint/1 -> OMAP_Module/53(JABSve_g_DbDecSetpoint)
  ICABve_d_ICAMode/1 -> OMAP_Module/96(ICABve_d_ICAMode)
  LKASve_y_Hands_Off_Warning/1 -> OMAP_Module/70(LKASve_y_Hands_Off_Warning)
  LKASve_y_LKA_Status_Display/1 -> OMAP_Module/68(LKASve_y_LKA_Status_Display)
  JABSve_d_DbAlertReq/1 -> OMAP_Module/62(JABSve_d_DbAlertReq)
  OMAP_Module/42(OMAPve_g_ADAS_LKAAngleReq) -> OMAPve_g_ADAS_LKAAngleReq/1
  OMAP_Module/40(OMAPve_y_ADAS_LKAState) -> OMAPve_y_ADAS_LKAState/1
  OMAP_Module/23(OMAPve_y_ADAS_ESCHoldReq) -> OMAPve_y_ADAS_ESCHoldReq/1
  AEBSve_d_JABS_HapticAlarm/1 -> OMAP_Module/49(AEBSve_d_JABS_HapticAlarm)
  OMAP_Module/45(OMAPve_g_ADAS_ESATorqueReq) -> OMAPve_g_ADAS_ESATorqueReq/1
  OMAP_Module/48(OMAPve_y_ADAS_ICAStatusIcon) -> OMAPve_y_ADAS_ICAStatusIcon/1
  OMAP_Module/17(OMAPve_y_ADAS_UpDownGearChange) -> OMAPve_y_ADAS_UpDownGearChange/1
  IMAPve_d_EPS_LKA_State/1 -> OMAP_Module/100(IMAPve_d_EPS_LKA_State)
  ACCSve_d_ACC_TqFlag/1 -> OMAP_Module/13(ACCSve_d_ACC_TqFlag)
  OMAP_Module/49(OMAPve_y_ADAS_HWAMode) -> OMAPve_y_ADAS_HWAMode/1
  FDMMve_d_EsaFcnConf/1 -> OMAP_Module/3(FDMMve_d_EsaFcnConf)
  IMAPve_g_R0_C2/1 -> OMAP_Module/111(IMAPve_g_R0_C2)
  OMAP_Module/24(OMAPve_y_ADAS_DecelerationType) -> OMAPve_y_ADAS_DecelerationType/1
  ACCSve_d_ACC_EPBReq/1 -> OMAP_Module/25(ACCSve_d_ACC_EPBReq)
  OMAP_Module/19(OMAPve_g_ADAS_DecelerationSet) -> OMAPve_g_ADAS_DecelerationSet/1
  AEBSve_d_AEBSwitchStatus/1 -> OMAP_Module/40(AEBSve_d_AEBSwitchStatus)
  JABSve_d_DbESCDriveOff/1 -> OMAP_Module/64(JABSve_d_DbESCDriveOff)
  OMAP_Module/35(OMAPve_y_ADAS_LKAStatusDisplay) -> OMAPve_y_ADAS_LKAStatusDisplay/1
  AEBSve_d_JABS_SwitchStatus/1 -> OMAP_Module/46(AEBSve_d_JABS_SwitchStatus)
  OMAP_Module/55(OMAPve_y_ADAS_State) -> OMAPve_y_ADAS_State/1
  OMAP_Module/51(OMAPve_y_ADAS_ESAFaultSt) -> OMAPve_y_ADAS_ESAFaultSt/1
  IMAPva_g_obj_pos_x/1 -> OMAP_Module/103(IMAPva_g_obj_pos_x)
  OMAP_Module/1(OMAPve_y_ADAS_ISLCState) -> OMAPve_y_ADAS_ISLCState/1
  ACCSve_d_SignalTStamp/1 -> OMAP_Module/21(ACCSve_d_SignalTStamp)
  FDMMve_d_LkaFcnConf/1 -> OMAP_Module/5(FDMMve_d_LkaFcnConf)
  OMAP_Module/46(OMAPve_y_ADAS_ESARequest) -> OMAPve_y_ADAS_ESARequest/1
  OMAP_Module/39(OMAPve_y_ADAS_LCAPopupMessage) -> OMAPve_y_ADAS_LCAPopupMessage/1
  ICABve_d_ICAState/1 -> OMAP_Module/97(ICABve_d_ICAState)
  ELKSve_y_Hands_Off_Warning/1 -> OMAP_Module/81(ELKSve_y_Hands_Off_Warning)
  AEBSve_d_ESCDriveOff/1 -> OMAP_Module/34(AEBSve_d_ESCDriveOff)
  ELKSve_y_ELK_HapticAlarmReq/1 -> OMAP_Module/80(ELKSve_y_ELK_HapticAlarmReq)
  ACCSve_d_HeadWaySet/1 -> OMAP_Module/20(ACCSve_d_HeadWaySet)
  LKASve_g_LKA_SWA_Control/1 -> OMAP_Module/74(LKASve_g_LKA_SWA_Control)
  ICABve_g_SteerAngleCmd/1 -> OMAP_Module/95(ICABve_g_SteerAngleCmd)
  IMAPve_g_L0_C3/1 -> OMAP_Module/108(IMAPve_g_L0_C3)
  FDMMve_d_JaFcnConf/1 -> OMAP_Module/1(FDMMve_d_JaFcnConf)
  FDMMve_d_SignalTStamp/1 -> OMAP_Module/10(FDMMve_d_SignalTStamp)
  ACCSve_d_ACC_State/1 -> OMAP_Module/11(ACCSve_d_ACC_State)
  LKASve_y_LKATorqueReq/1 -> OMAP_Module/77(LKASve_y_LKATorqueReq)
  LKASve_g_LKATorqueReq_Value/1 -> OMAP_Module/78(LKASve_g_LKATorqueReq_Value)
  ELKSve_y_LKATorqueReq/1 -> OMAP_Module/91(ELKSve_y_LKATorqueReq)
  ELKSve_g_LKATorqueReq_Value/1 -> OMAP_Module/92(ELKSve_g_LKATorqueReq_Value)
  ICABve_d_LKATorqueReq/1 -> OMAP_Module/98(ICABve_d_LKATorqueReq)
  ICABve_g_LKATorqueReq_Value/1 -> OMAP_Module/99(ICABve_g_LKATorqueReq_Value)
  IMAPve_d_APA_AutoPark_WorkSt/1 -> OMAP_Module/113(IMAPve_d_APA_AutoPark_WorkSt)
  OMAP_Module/57(OMAPve_g_ob019L_100) -> OMAPve_g_ob019L_100/1
  ACCSve_d_ACC_ISLCState/1 -> OMAP_Module/27(ACCSve_d_ACC_ISLCState)
  ACCSve_d_ACC_ISLCDriverRemind/1 -> OMAP_Module/28(ACCSve_d_ACC_ISLCDriverRemind)
  OMAP_Module/58(OMAPve_y_ADAS_ELKPopupMessage) -> OMAPve_y_ADAS_ELKPopupMessage/1
  OMAP_Module/59(OMAPve_y_ADAS_TurnLightsCommand) -> OMAPve_y_ADAS_TurnLightsCommand/1
  ESASve_y_ESA_State/1 -> OMAP_Module/114(ESASve_y_ESA_State)
  ESASve_g_ESA_SWA_CMD/1 -> OMAP_Module/115(ESASve_g_ESA_SWA_CMD)
  ESASve_g_EPS_Factor_Control/1 -> OMAP_Module/116(ESASve_g_EPS_Factor_Control)
  ESASve_y_ESA_FaultSt/1 -> OMAP_Module/117(ESASve_y_ESA_FaultSt)
  ESASve_y_ESARequest/1 -> OMAP_Module/118(ESASve_y_ESARequest)
  ESASve_y_ESATorqueReq/1 -> OMAP_Module/119(ESASve_y_ESATorqueReq)
  ESASve_y_LKAActivation/1 -> OMAP_Module/120(ESASve_y_LKAActivation)
  ACCSve_d_ACCMessagePrompt/1 -> OMAP_Module/26(ACCSve_d_ACCMessagePrompt)
